simulink model "furutaPend_fcn"  (R2017b)
settings: Solver=VariableStepAuto  StartTime=0.0  StopTime=10.0  RelTol=1e-3
settings Model: Creator=ozhanyz  LastModifiedBy=ozhanyz

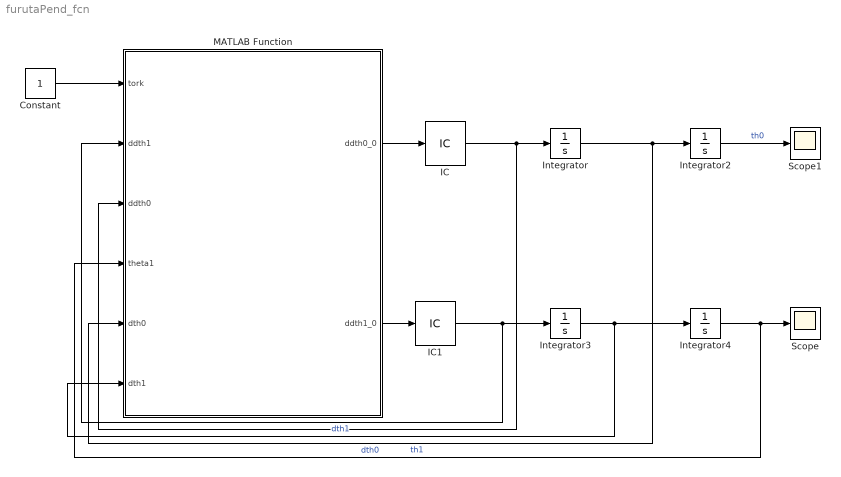
== system furutaPend_fcn ==
  Constant : Constant
  IC : InitialCondition  Value=0.0000001
  IC1 : InitialCondition  Value=0.0000001
  Integrator{,2..4} (4 alike) : Integrator
  MATLAB Function : MATLAB Function  TreatAsAtomicUnit=on
  Scope : Scope
  Scope1 : Scope
  wires:
  Integrator/1 -> MATLAB Function/5(dth0), Integrator2/1  "dth0"
  Integrator3/1 -> MATLAB Function/6(dth1), Integrator4/1  "dth1"
  MATLAB Function/2(ddth1_0) -> IC1/1
  Integrator4/1 -> MATLAB Function/4(theta1), Scope/1  "th1"
  Integrator2/1 -> Scope1/1  "th0"
  MATLAB Function/1(ddth0_0) -> IC/1
  Constant/1 -> MATLAB Function/1(tork)
  IC/1 -> MATLAB Function/3(ddth0), Integrator/1
  IC1/1 -> MATLAB Function/2(ddth1), Integrator3/1

== matlab function furutaPend_fcn/MATLAB Function ==
  data: tork input; ddth0_0 output; ddth1 input; ddth0 input; theta1 input; dth0 input; dth1 input; ddth1_0 output
function[ddth0_0,ddth1_0] = fcn(tork,ddth1,ddth0,theta1,dth0,dth1)
m=5.38*10^(-2);     Io=1.75*10^(-2);    Lo=0.215;
L1=0.25;        l1=0.113;       J1=1.98*10^(-4);
g=9.81;




ddth0_0=(tork-m*l1*(Lo*cos(theta1)*ddth1+l1*sin(2*theta1)*dth0*dth1-Lo*sin(theta1)*dth1*dth1))/(Io+m*Lo*Lo+l1*l1*m*sin(theta1)*sin(theta1))

ddth1_0=m*l1*(l1*sin(theta1)*cos(theta1)*(dth0^2)+g*sin(theta1)-Lo*cos(theta1)*dth0)/(J1+m*l1*l1)
